simulink model "DrvStRclCmdSrvCal"  (R2018b)
settings: Solver=FixedStepDiscrete  StartTime=0.0  StopTime=10.0  FixedStep=0.01  RelTol=1e-3
undefined symbols (not defined in the file or in its folder): KeSMSwPosInvalidVal_Val, PowerMode1
settings Model: Creator=sn2xws  LastModifiedBy=sn2xws
settings DataIOCC: SaveFormat=StructureWithTime
settings OptimizationCC: DefaultParameterBehavior=Inlined  EnhancedBackFolding=on  PassReuseOutputArgsAs=Individual arguments  ZeroExternalMemoryAtStartup=off  ZeroInternalMemoryAtStartup=off  OptimizeBlockOrder=speed  DifferentSizesBufferReuse=on  OptimizationCustomize=off
settings DebuggingCC: ParameterTunabilityLossMsg=error
settings ModelReferenceCC: ModelReferenceNumInstancesAllowed=Single
settings SFSimCC: MATLABDynamicMemAlloc=off
settings RTWCC: SystemTargetFile=autosar.tlc  GenCodeOnly=on  TemplateMakefile=ert_default_tmf  Description=AUTOSAR  GenerateReport=on  IncludeHyperlinkInReport=on  LaunchReport=on  GenerateTraceInfo=on  GenerateTraceReport=on  GenerateTraceReportSl=on  GenerateTraceReportSf=on  GenerateTraceReportEml=on  GenerateCodeMetricsReport=on
settings CodeAppCC: ForceParamTrailComments=on  IgnoreCustomStorageClasses=off  OperatorAnnotations=on  SimulinkDataObjDesc=on  SFDataObjDesc=on  InsertBlockDesc=on
settings STFCustomTargetCC: TargetLangStandard=C99 (ISO)  MultiwordLength=256  ParMdlRefBuildCompliant=on  CompOptLevelCompliant=on  IncludeMdlTerminateFcn=off  CombineOutputUpdateFcns=on  SuppressErrorStatus=on  ERTCustomFileBanners=on  SupportNonFinite=off  SupportComplex=off  SupportContinuousTime=off  SupportNonInlinedSFcns=off  RemoveResetFunc=on  MATLABClassNameForMDSCustomization=Simulink.SoftwareTarget.ERTCustomization  AutosarCompliant=on  UseToolchainInfoCompliant=on  LookupTableObjectStructAxisOrder=2,1,3,4,...  LUTObjectStructOrderEvenSpacing=Size,Table,Breakpoints  SystemTargetFile=autosar.tlc
settings ERTTargetCC: TargetLangStandard=C99 (ISO)  ConcurrentExecutionCompliant=off  IncludeMdlTerminateFcn=off  SuppressErrorStatus=on  SupportNonFinite=off  SupportComplex=off  ModelStepFunctionPrototypeControlCompliant=off  CPPClassGenCompliant=off  AutosarCompliant=on  LookupTableObjectStructAxisOrder=2,1,3,4,...  LUTObjectStructOrderEvenSpacing=Size,Table,Breakpoints  InlinedParameterPlacement=NonHierarchical  ERTCustomFileTemplate=example_file_process.tlc  ERTFilePackagingFormat=Compact

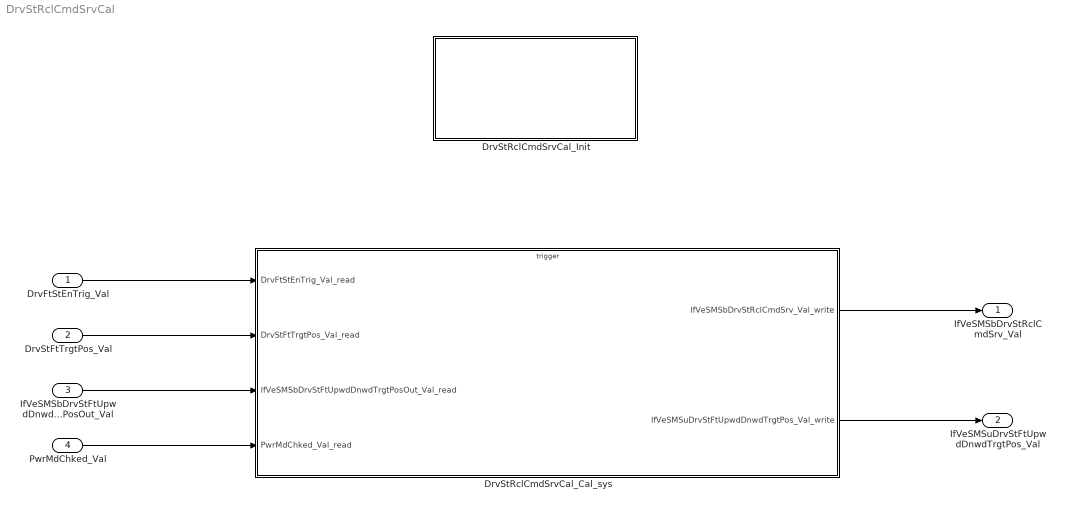
== system DrvStRclCmdSrvCal ==
  DrvFtStEnTrig_Val : Inport  OutDataTypeStr=boolean  PortDimensions=1
  DrvStFtTrgtPos_Val : Inport  Port=2  OutDataTypeStr=uint16  PortDimensions=1
  IfVeSMSbDrvStFtUpwdDnwdTrgtPosOut_Val : Inport  Port=3  OutDataTypeStr=boolean  PortDimensions=1
  PwrMdChked_Val : Inport  Port=4  OutDataTypeStr=Enum: PowerMode1  PortDimensions=1
  DrvStRclCmdSrvCal_Cal_sys : Subsystem
  DrvStRclCmdSrvCal_Init : Subsystem
  IfVeSMSbDrvStRclCmdSrv_Val : Outport  OutDataTypeStr=boolean  PortDimensions=1
  IfVeSMSuDrvStFtUpwdDnwdTrgtPos_Val : Outport  Port=2  OutDataTypeStr=uint16  PortDimensions=1
  wires:
  DrvStRclCmdSrvCal_Cal_sys/1(IfVeSMSbDrvStRclCmdSrv_Val_write) -> IfVeSMSbDrvStRclCmdSrv_Val/1
  DrvStRclCmdSrvCal_Cal_sys/2(IfVeSMSuDrvStFtUpwdDnwdTrgtPos_Val_write) -> IfVeSMSuDrvStFtUpwdDnwdTrgtPos_Val/1
  DrvFtStEnTrig_Val/1 -> DrvStRclCmdSrvCal_Cal_sys/1(DrvFtStEnTrig_Val_read)
  DrvStFtTrgtPos_Val/1 -> DrvStRclCmdSrvCal_Cal_sys/2(DrvStFtTrgtPos_Val_read)
  IfVeSMSbDrvStFtUpwdDnwdTrgtPosOut_Val/1 -> DrvStRclCmdSrvCal_Cal_sys/3(IfVeSMSbDrvStFtUpwdDnwdTrgtPosOut_Val_read)
  PwrMdChked_Val/1 -> DrvStRclCmdSrvCal_Cal_sys/4(PwrMdChked_Val_read)

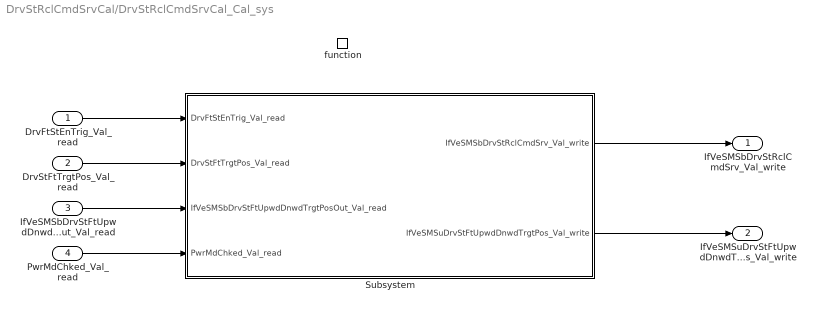
== system DrvStRclCmdSrvCal/DrvStRclCmdSrvCal_Cal_sys ==
  DrvFtStEnTrig_Val_read : Inport
  DrvStFtTrgtPos_Val_read : Inport  Port=2
  IfVeSMSbDrvStFtUpwdDnwdTrgtPosOut_Val_read : Inport  Port=3
  PwrMdChked_Val_read : Inport  Port=4
  function : TriggerPort  TriggerType=function-call  IsSimulinkFunction=on  FunctionName=DrvStRclCmdSrvCal_Cal  VariantControl=(inherit)
  Subsystem : Subsystem
  IfVeSMSbDrvStRclCmdSrv_Val_write : Outport
      settings: EnsureOutportIsVirtual=on
  IfVeSMSuDrvStFtUpwdDnwdTrgtPos_Val_write : Outport  Port=2
      settings: EnsureOutportIsVirtual=on
  wires:
  DrvFtStEnTrig_Val_read/1 -> Subsystem/1(DrvFtStEnTrig_Val_read)
  DrvStFtTrgtPos_Val_read/1 -> Subsystem/2(DrvStFtTrgtPos_Val_read)
  IfVeSMSbDrvStFtUpwdDnwdTrgtPosOut_Val_read/1 -> Subsystem/3(IfVeSMSbDrvStFtUpwdDnwdTrgtPosOut_Val_read)
  Subsystem/1(IfVeSMSbDrvStRclCmdSrv_Val_write) -> IfVeSMSbDrvStRclCmdSrv_Val_write/1
  Subsystem/2(IfVeSMSuDrvStFtUpwdDnwdTrgtPos_Val_write) -> IfVeSMSuDrvStFtUpwdDnwdTrgtPos_Val_write/1
  PwrMdChked_Val_read/1 -> Subsystem/4(PwrMdChked_Val_read)

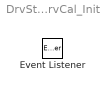
== system DrvStRclCmdSrvCal/DrvStRclCmdSrvCal_Init ==
  Event Listener : EventListener  EventName=reset

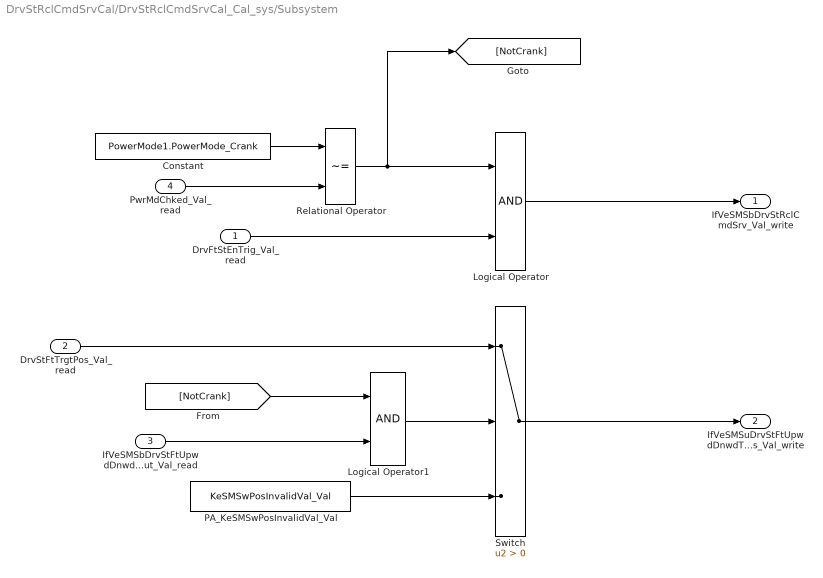
== system DrvStRclCmdSrvCal/DrvStRclCmdSrvCal_Cal_sys/Subsystem ==
  DrvFtStEnTrig_Val_read : Inport
  DrvStFtTrgtPos_Val_read : Inport  Port=2
  IfVeSMSbDrvStFtUpwdDnwdTrgtPosOut_Val_read : Inport  Port=3
  PwrMdChked_Val_read : Inport  Port=4
  Constant : Constant  Value=PowerMode1.PowerMode_Crank  OutDataTypeStr=Enum: PowerMode1
  Logical Operator : Logic  AllPortsSameDT=off  OutDataTypeStr=boolean
  Logical Operator1 : Logic  AllPortsSameDT=off  OutDataTypeStr=boolean
  PA_KeSMSwPosInvalidVal_Val : Constant  Value=KeSMSwPosInvalidVal_Val
  Relational Operator : RelationalOperator  Operator=~=  OutDataTypeStr=boolean  RndMeth=Simplest
  Switch : Switch  Criteria=u2 > Threshold
  IfVeSMSbDrvStRclCmdSrv_Val_write : Outport
      settings: EnsureOutportIsVirtual=on
  IfVeSMSuDrvStFtUpwdDnwdTrgtPos_Val_write : Outport  Port=2
      settings: EnsureOutportIsVirtual=on
  wires:
  Switch/1 -> IfVeSMSuDrvStFtUpwdDnwdTrgtPos_Val_write/1
  Logical Operator/1 -> IfVeSMSbDrvStRclCmdSrv_Val_write/1
  DrvFtStEnTrig_Val_read/1 -> Logical Operator/2
  DrvStFtTrgtPos_Val_read/1 -> Switch/1
  PA_KeSMSwPosInvalidVal_Val/1 -> Switch/3
  PwrMdChked_Val_read/1 -> Relational Operator/2
  Constant/1 -> Relational Operator/1
  Relational Operator/1 -> [NotCrank], Logical Operator/1
  Logical Operator1/1 -> Switch/2
  IfVeSMSbDrvStFtUpwdDnwdTrgtPosOut_Val_read/1 -> Logical Operator1/2
  [NotCrank] -> Logical Operator1/1
